simulink model "chap2_4"  (Simulink 3.00)
settings: Solver=ode45  StartTime=0.0  StopTime=2000  RelTol=1e-3
libraries: simulink_extras x1

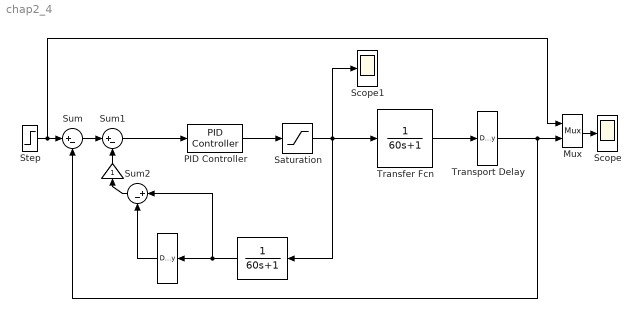
== system chap2_4 ==
  " " : Gain  Orientation=up  Gain=1  SaturateOnIntegerOverflow=on
  "  " : TransportDelay  Orientation=left  DelayTime=80  InitialInput=0  BufferSize=1024
  "    " : TransferFcn  Orientation=left  Numerator=[1]  Denominator=[60 1]
  Mux : Mux  Inputs=2
      settings: DisplayOption=none
  PID Controller : simulink_extras/Additional Linear/PID Controller  P=4  I=0.022  D=0.0
  Saturation : Saturate  UpperLimit=110  LowerLimit=-110
  Scope : Scope
      settings: TimeRange=auto  YMin=-1  YMax=1  SaveToWorkspace=off  SaveName=ScopeData
  Scope1 : Scope
      settings: TimeRange=auto  YMin=-1  YMax=1  SaveToWorkspace=off  SaveName=ScopeData
  Step : Step  Time=0  Before=0  After=100  SampleTime=20
  Sum : Sum  Inputs=|+-  SaturateOnIntegerOverflow=on
  Sum1 : Sum  Inputs=|+-  SaturateOnIntegerOverflow=on
  Sum2 : Sum  Orientation=left  Inputs=|+-  SaturateOnIntegerOverflow=on
  Transfer Fcn : TransferFcn  Numerator=[1]  Denominator=[60 1]
  Transport Delay : TransportDelay  DelayTime=80  InitialInput=0  BufferSize=1024
  wires:
  PID Controller/1 -> Saturation/1
  Saturation/1 -> Transfer Fcn/1, "    "/1, Scope1/1
  "    "/1 -> Sum2/1, "  "/1
  Sum/1 -> Sum1/1
  Step/1 -> Sum/1, Mux/1
  Sum1/1 -> PID Controller/1
  " "/1 -> Sum1/2
  "  "/1 -> Sum2/2
  Sum2/1 -> " "/1
  Transfer Fcn/1 -> Transport Delay/1
  Transport Delay/1 -> Mux/2, Sum/2
  Mux/1 -> Scope/1
